simulink model "APPL_DriverFaultDetection"  (R2018b)
settings: configuration reference "CodeConfig_10_ms" (kept outside this file)
undefined symbols (not defined in the file): CAL_LockErrNoTime_30ms, CAL_ManualSwValid_90s, CAL_MotorHallInvalid_2s, CAL_MotorMaxRunTime_60s, CAL_MotorRelayErr_2s, CAL_MotorStall_750ms, D_DrSoftStopDef_B, D_DrSoftStopDef_F, D_DrSoftStopDef_H, D_DrSoftStopDef_L, D_Relay_DownBackFault, D_Relay_UpFrontFault, enSeatMoveCmd, FALSE, TRUE
libraries: DareLib x95, simulink x2
(part 3 of 3)

== stateflow chart APPL_DriverFaultDetection/LogicCtrl/HallError/HallErrorDetection ==
  note: #后期需要增加2F诊断判断20230510
  state MotorHallDetect
    state HeightHallError [parallel]
      settings: executionOrder=1
      state Judge
        ex:
        HeightHallTimer = 0;
        (default) -> (junction 16)
        MotorHallDetect.HeightHallError.Judge -> (junction 16) [order 1]
        (junction 16) -> (junction 19) [order 1] : /*2s超时检测*/
            | [CAL_MotorHallInvalid_2s > HeightHallTimer]
        (junction 19) -> (junction 178)
        (junction 16) -> (junction 30) [order 2] : {HeightHallTimer = CAL_MotorHallInvalid_2s;
            | HeightHallFault = 1;
            | Desc_HeightHallDTC = 1;}
        (junction 178) -> (junction 180) [order 1] : /* 粘连或无电机动作 */
            | [MtrCtrlFault_HeightUpVolt == MtrCtrlFault_HeightDownVolt ...
            | || enSeatMoveCmd.EN_NULL == MtrCtrlFault_HeightMotorCmd]
        (junction 178) -> (junction 162) [order 2] : {HeightHallTimer ++;}
        (junction 180) -> (junction 182) : {HeightHallTimer = 0;}
        (junction 162) -> (junction 30)
        (junction 182) -> (junction 162)
        (junction 30) -> (junction 21)
        (junction 21) -> (junction 23) [order 1] : /*霍尔计数变化*/
            | [hasChanged(MtrCtrlFault_HeightHallCnt)]
        (junction 21) -> (junction 28) [order 2]
        (junction 23) -> (junction 26) : {HeightHallTimer = 0;
            | HeightHallFault = 0;
            | Desc_HeightHallDTC = 0;}
        (junction 26) -> (junction 28)
      state Normal
        en:
        HeightHallFault = 0;
      state Init
        en:
        HeightHallFault = 0;
        Desc_HeightHallDTC = 0;
      (default) -> MotorHallDetect.HeightHallError.Normal
      MotorHallDetect.HeightHallError.Normal -> MotorHallDetect.HeightHallError.Judge [order 2] : /*有调节动作*/
          | [enSeatMoveCmd.EN_NULL != MtrCtrlFault_HeightMotorCmd]
      MotorHallDetect.HeightHallError.Judge -> MotorHallDetect.HeightHallError.Normal [order 2] : /* */
          | [(hasChanged(HeightSwCmd) ...
          | || enSeatMoveCmd.EN_NULL == HeightSwCmd) ...
          | && enSeatMoveCmd.EN_NULL == MtrCtrlFault_HeightMotorCmd]
      MotorHallDetect.HeightHallError.Judge -> MotorHallDetect.HeightHallError.Init [order 1] : /* 不满足前置条件 */
          | [FALSE == DrAdj_Dtc_HeatingMat1SC]
      MotorHallDetect.HeightHallError.Init -> MotorHallDetect.HeightHallError.Normal : /* 满足前置条件 */
          | [TRUE == DrAdj_Dtc_HeatingMat1SC]
      MotorHallDetect.HeightHallError.Normal -> MotorHallDetect.HeightHallError.Init [order 1] : /* 不满足前置条件 */
          | [FALSE == DrAdj_Dtc_HeatingMat1SC]
    state LengthHallError [parallel]
      settings: executionOrder=2
      state Normal
        en:
        LengthHallFault = 0;
      state Judge
        ex:
        LengthHallTimer = 0;
        (default) -> (junction 53)
        MotorHallDetect.LengthHallError.Judge -> (junction 53) [order 1]
        (junction 53) -> (junction 57) [order 1] : /*2s超时检测*/
            | [CAL_MotorHallInvalid_2s > LengthHallTimer]
        (junction 53) -> (junction 68) [order 2] : {LengthHallTimer = CAL_MotorHallInvalid_2s;
            | LengthHallFault = 1;
            | Desc_LengthHallDTC = 1;}
        (junction 57) -> (junction 185)
        (junction 185) -> (junction 187) [order 1] : /*粘连或无电机动作*/
            | [MtrCtrlFault_LengthForwardVolt == MtrCtrlFault_LengthBackwardVolt ...
            | || enSeatMoveCmd.EN_NULL == MtrCtrlFault_LengthMotorCmd]
        (junction 185) -> (junction 164) [order 2] : {LengthHallTimer ++;}
        (junction 187) -> (junction 189) : {LengthHallTimer = 0;}
        (junction 164) -> (junction 68)
        (junction 189) -> (junction 164)
        (junction 68) -> (junction 60)
        (junction 60) -> (junction 52) [order 1] : /*霍尔计数变化*/
            | [hasChanged(MtrCtrlFault_LengthHallCnt)]
        (junction 60) -> (junction 74) [order 2]
        (junction 52) -> (junction 62) : {LengthHallTimer = 0;
            | LengthHallFault = 0;
            | Desc_LengthHallDTC = 0;}
        (junction 62) -> (junction 74)
        (junction 74) -> (junction 64)
      state Init
        en:
        LengthHallFault = 0;
        Desc_LengthHallDTC = 0;
      (default) -> MotorHallDetect.LengthHallError.Normal
      MotorHallDetect.LengthHallError.Normal -> MotorHallDetect.LengthHallError.Judge [order 2] : /*有调节动作*/
          | [enSeatMoveCmd.EN_NULL != MtrCtrlFault_LengthMotorCmd]
      MotorHallDetect.LengthHallError.Judge -> MotorHallDetect.LengthHallError.Normal [order 2] : /*无调节动作*/
          | [(hasChanged(LengthSwCmd) ...
          | || enSeatMoveCmd.EN_NULL == LengthSwCmd) ...
          | && enSeatMoveCmd.EN_NULL == MtrCtrlFault_LengthMotorCmd]
      MotorHallDetect.LengthHallError.Judge -> MotorHallDetect.LengthHallError.Init [order 1] : /* 不满足前置条件 */
          | [FALSE == DrAdj_Dtc_HeatingMat1SC]
      MotorHallDetect.LengthHallError.Init -> MotorHallDetect.LengthHallError.Normal : /* 满足前置条件 */
          | [TRUE == DrAdj_Dtc_HeatingMat1SC]
      MotorHallDetect.LengthHallError.Normal -> MotorHallDetect.LengthHallError.Init [order 1] : /* 不满足前置条件 */
          | [FALSE == DrAdj_Dtc_HeatingMat1SC]
    state BackHallError [parallel]
      settings: executionOrder=3
      state Judge
        ex:
        BackHallTimer = 0;
        (default) -> (junction 87)
        MotorHallDetect.BackHallError.Judge -> (junction 87) [order 1]
        (junction 87) -> (junction 91) [order 1] : /*2s超时检测*/
            | [CAL_MotorHallInvalid_2s > BackHallTimer]
        (junction 87) -> (junction 102) [order 2] : {BackHallTimer = CAL_MotorHallInvalid_2s;
            | BackHallFault = 1;
            | Desc_BackHallDTC = 1;}
        (junction 91) -> (junction 192)
        (junction 192) -> (junction 194) [order 1] : /*粘连或无电机动作*/
            | [MtrCtrlFault_BackForwardVolt == MtrCtrlFault_BackBackwardVolt ...
            | || enSeatMoveCmd.EN_NULL == MtrCtrlFault_BackMotorCmd]
        (junction 192) -> (junction 166) [order 2] : {BackHallTimer ++;}
        (junction 194) -> (junction 196) : {BackHallTimer = 0;}
        (junction 166) -> (junction 102)
        (junction 196) -> (junction 166)
        (junction 102) -> (junction 94)
        (junction 94) -> (junction 86) [order 1] : /*霍尔计数变化*/
            | [hasChanged(MtrCtrlFault_BackHallCnt)]
        (junction 94) -> (junction 108) [order 2]
        (junction 86) -> (junction 96) : {BackHallTimer = 0;
            | BackHallFault = 0;
            | Desc_BackHallDTC = 0;}
        (junction 96) -> (junction 108)
        (junction 108) -> (junction 98)
      state Normal
        en:
        BackHallFault = 0;
      state Init
        en:
        BackHallFault = 0;
        Desc_BackHallDTC = 0;
      (default) -> MotorHallDetect.BackHallError.Normal
      MotorHallDetect.BackHallError.Normal -> MotorHallDetect.BackHallError.Judge [order 2] : /*有调节动作*/
          | [enSeatMoveCmd.EN_NULL != MtrCtrlFault_BackMotorCmd]
      MotorHallDetect.BackHallError.Judge -> MotorHallDetect.BackHallError.Normal [order 2] : /*无调节动作*/
          | [(hasChanged(BackSwCmd) ...
          | || enSeatMoveCmd.EN_NULL == BackSwCmd) ...
          | && enSeatMoveCmd.EN_NULL == MtrCtrlFault_BackMotorCmd]
      MotorHallDetect.BackHallError.Judge -> MotorHallDetect.BackHallError.Init [order 1] : /* 不满足前置条件 */
          | [FALSE == DrAdj_Dtc_HeatingMat1SC]
      MotorHallDetect.BackHallError.Init -> MotorHallDetect.BackHallError.Normal : /* 满足前置条件 */
          | [TRUE == DrAdj_Dtc_HeatingMat1SC]
      MotorHallDetect.BackHallError.Normal -> MotorHallDetect.BackHallError.Init [order 1] : /* 不满足前置条件 */
          | [FALSE == DrAdj_Dtc_HeatingMat1SC]
    state FrontHallError3 [parallel]
      settings: executionOrder=4
      state Judge
        ex:
        FrontHallTimer = 0;
        (default) -> (junction 121)
        MotorHallDetect.FrontHallError3.Judge -> (junction 121) [order 1]
        (junction 121) -> (junction 125) [order 1] : /*2s超时检测*/
            | [CAL_MotorHallInvalid_2s > FrontHallTimer]
        (junction 121) -> (junction 136) [order 2] : {FrontHallTimer = CAL_MotorHallInvalid_2s;
            | FrontHallFault = 1;
            | Desc_FrontHallDTC = 1;}
        (junction 125) -> (junction 199)
        (junction 199) -> (junction 201) [order 1] : /*粘连或无电机动作*/
            | [MtrCtrlFault_FrontUpVolt == MtrCtrlFault_FrontDownVolt ...
            | || enSeatMoveCmd.EN_NULL == MtrCtrlFault_FrontMotorCmd]
        (junction 199) -> (junction 169) [order 2] : {FrontHallTimer ++;}
        (junction 201) -> (junction 203) : {FrontHallTimer = 0;}
        (junction 169) -> (junction 136)
        (junction 203) -> (junction 169)
        (junction 136) -> (junction 128)
        (junction 128) -> (junction 120) [order 1] : /*霍尔计数变化*/
            | [hasChanged(MtrCtrlFault_FrontHallCnt)]
        (junction 128) -> (junction 142) [order 2]
        (junction 120) -> (junction 130) : {FrontHallTimer = 0;
            | FrontHallFault = 0;
            | Desc_FrontHallDTC = 0;}
        (junction 130) -> (junction 142)
        (junction 142) -> (junction 132)
      state Normal
        en:
        FrontHallFault = 0;
      state Init
        en:
        FrontHallFault = 0;
        Desc_FrontHallDTC = 0;
      (default) -> MotorHallDetect.FrontHallError3.Normal
      MotorHallDetect.FrontHallError3.Normal -> MotorHallDetect.FrontHallError3.Judge [order 1] : /*有调节动作*/
          | [enSeatMoveCmd.EN_NULL != MtrCtrlFault_FrontMotorCmd ...
          |  && EN_DrTwelveWayMotor == MtrCtrlFault_DrAdjustCfg]
      MotorHallDetect.FrontHallError3.Judge -> MotorHallDetect.FrontHallError3.Normal [order 2] : /*无调节动作*/
          | [((hasChanged(FrontSwCmd) ...
          | || enSeatMoveCmd.EN_NULL == FrontSwCmd) ...
          | && enSeatMoveCmd.EN_NULL == MtrCtrlFault_FrontMotorCmd) ...
          | || EN_DrTwelveWayMotor != MtrCtrlFault_DrAdjustCfg]
      MotorHallDetect.FrontHallError3.Init -> MotorHallDetect.FrontHallError3.Normal : /* 满足前置条件 */
          | [TRUE == DrAdj_Dtc_HeatingMat1SC]
      MotorHallDetect.FrontHallError3.Judge -> MotorHallDetect.FrontHallError3.Init [order 1] : /* 不满足前置条件 */
          | [FALSE == DrAdj_Dtc_HeatingMat1SC ...
          | || EN_DrTwelveWayMotor != MtrCtrlFault_DrAdjustCfg]
      MotorHallDetect.FrontHallError3.Normal -> MotorHallDetect.FrontHallError3.Init [order 2] : /* 不满足前置条件 */
          | [FALSE == DrAdj_Dtc_HeatingMat1SC]
  state Init
    en:
    HeightHallFault = 0;
    HeightHallTimer = 0;
    Desc_HeightHallDTC = 0;
    LengthHallFault = 0;
    LengthHallTimer = 0;
    Desc_LengthHallDTC = 0;
    BackHallFault = 0;
    BackHallTimer = 0;
    Desc_BackHallDTC = 0;
    FrontHallFault = 0;
    FrontHallTimer = 0;
    Desc_FrontHallDTC = 0;
  (default) -> Init
  Init -> MotorHallDetect : /* 有记忆功能 且非不可调节配置 */
      | [TRUE == MtrCtrlFault_DrMemoryCfg ...
      | && (EN_DrSixWayMotor == MtrCtrlFault_DrAdjustCfg ...
      |     || EN_DrTwelveWayMotor == MtrCtrlFault_DrAdjustCfg)]
  MotorHallDetect -> Init : /* 无记忆功能 ||不可调节配置 */
      | [TRUE != MtrCtrlFault_DrMemoryCfg ...
      | || (EN_DrSixWayMotor != MtrCtrlFault_DrAdjustCfg ...
      |     && EN_DrTwelveWayMotor != MtrCtrlFault_DrAdjustCfg)]
  data: HeightSwCmd input; LengthSwCmd input; BackSwCmd input; FrontSwCmd input; MtrCtrlFault_HeightUpVolt input; MtrCtrlFault_HeightDownVolt input; MtrCtrlFault_LengthForwardVolt input; MtrCtrlFault_LengthBackwardVolt input; Desc_HeightHallDTC output uint8 =0; Desc_LengthHallDTC output uint8 =0; Desc_BackHallDTC output uint8 =0; Desc_FrontHallDTC output uint8 =0; MtrCtrlFault_BackForwardVolt input; MtrCtrlFault_BackBackwardVolt input; MtrCtrlFault_FrontUpVolt input; MtrCtrlFault_FrontDownVolt input; HeightHallFault output uint8; MtrCtrlFault_HeightHallCnt input; MtrCtrlFault_LengthHallCnt input; MtrCtrlFault_BackHallCnt input; MtrCtrlFault_FrontHallCnt input; MtrCtrlFault_HeightMotorCmd input; MtrCtrlFault_LengthMotorCmd input; MtrCtrlFault_BackMotorCmd input; MtrCtrlFault_FrontMotorCmd input; HeightHallTimer local uint8; CAL_MotorHallInvalid_2s parameter; LengthHallTimer local uint8; LengthHallFault output uint8; BackHallTimer local uint8; BackHallFault output uint8; FrontHallTimer local uint8; FrontHallFault output uint8; FALSE parameter; TRUE parameter; DrAdj_Dtc_HeatingMat1SC local boolean =1; MtrCtrlFault_DrAdjustCfg input; MtrCtrlFault_DrMemoryCfg input

== stateflow chart APPL_DriverFaultDetection/LogicCtrl/StallError/StallErrorDetection ==
  state HeightStallError [parallel]
    settings: executionOrder=1
    state Judge
      ex:
      HeightStallTimer = 0;
      HeightStallNoTimer = 0;
      (default) -> (junction 16)
      HeightStallError.Judge -> (junction 16) [order 1]
      (junction 16) -> (junction 19) [order 1] : /*达到堵转电流 且无霍尔变化 */
          | [LocalHeightHallCnt == MtrCtrlFault_HeightHallCnt]
      (junction 19) -> (junction 187) [order 1] : [1 == MtrCtrlFault_HeightCurrentOverFlag]
      (junction 187) -> (junction 194) [order 1] : [CurrentOverTimer1 < 255]
      (junction 16) -> (junction 30) [order 2] : {HeightStallTimer = 0;
          | CurrentOverTimer1 = 0;}
      (junction 19) -> (junction 191) [order 2] : {CurrentOverTimer1 = 0;}
      (junction 187) -> (junction 189) [order 2]
      (junction 194) -> (junction 196) : /* 高度大电流计时器 - 启动电压不超过30ms*/
          | {CurrentOverTimer1 ++;}
      (junction 189) -> (junction 191)
      (junction 196) -> (junction 189)
      (junction 191) -> (junction 21)
      (junction 21) -> (junction 23) [order 1] : /*高度的堵转条件检测*/
          | [HeightStallTimer > CAL_MotorStall_750ms  ...
          | && CurrentOverTimer1 > 20]
      (junction 21) -> (junction 28) [order 2] : /* 高度无霍尔计时器*/
          | {HeightStallTimer ++;}
      (junction 23) -> (junction 26) : {HeightStallFault = 1;
          | HeightStallTimer = CAL_MotorStall_750ms;
          | HeightStallNoTimer = 0;}
      (junction 28) -> (junction 30)
      (junction 26) -> (junction 28)
      (junction 30) -> (junction 43) : {LocalHeightHallCnt = MtrCtrlFault_HeightHallCnt;}
      (junction 43) -> (junction 161) [order 1] : /*无调节动作 同时没有本地开关*/
          | [enSeatMoveCmd.EN_NULL == MtrCtrlFault_HeightMotorCmd ...
          | && enSeatMoveCmd.EN_NULL == HeightSwCmd]
      (junction 43) -> (junction 169) [order 2]
      (junction 161) -> (junction 163) : {HeightStallNoTimer++;}
      (junction 163) -> (junction 169)
      (junction 169) -> (junction 172)
    state Normal
      en:
      HeightStallFault = 0;
      CurrentOverTimer1 = 0;
    (default) -> HeightStallError.Normal
    HeightStallError.Normal -> HeightStallError.Judge : /*有调节动作*/
        | [enSeatMoveCmd.EN_NULL != MtrCtrlFault_HeightMotorCmd ...
        | && MtrCtrl_PowerModeStatus != enIgnSts.eCrank]
    HeightStallError.Judge -> HeightStallError.Normal [order 1] : /* 超过故障计时 或按键变化 */
        | [CAL_LockErrNoTime_30ms < HeightStallNoTimer ...
        | || hasChanged(HeightSwCmd) ...
        | || MtrCtrl_PowerModeStatus == enIgnSts.eCrank]
  state LengthStallError [parallel]
    settings: executionOrder=2
    state Judge
      ex:
      LengthStallTimer = 0;
      LengthStallNoTimer = 0;
      (default) -> (junction 53)
      LengthStallError.Judge -> (junction 53) [order 1]
      (junction 53) -> (junction 57) [order 1] : /*达到堵转电流 且无霍尔变化*/
          | [LocalLengthHallCnt == MtrCtrlFault_LengthHallCnt]
      (junction 57) -> (junction 210) [order 1] : [1 == MtrCtrlFault_LengthCurrentOverFlag]
      (junction 210) -> (junction 212) [order 1] : [CurrentOverTimer2 < 255]
      (junction 53) -> (junction 68) [order 2] : {LengthStallTimer = 0;
          | CurrentOverTimer2 = 0;}
      (junction 57) -> (junction 208) [order 2] : {CurrentOverTimer2 = 0;}
      (junction 210) -> (junction 216) [order 2]
      (junction 212) -> (junction 214) : /* 纵向大电流计时器*/
          | {CurrentOverTimer2 ++;}
      (junction 216) -> (junction 208)
      (junction 214) -> (junction 216)
      (junction 208) -> (junction 60)
      (junction 60) -> (junction 52) [order 1] : /*纵向的堵转条件检测*/
          | [LengthStallTimer > CAL_MotorStall_750ms  ...
          | && CurrentOverTimer2 > 20]
      (junction 60) -> (junction 74) [order 2] : {LengthStallTimer ++;}
      (junction 52) -> (junction 62) : {LengthStallTimer = CAL_MotorStall_750ms;
          | LengthStallFault = 1;
          | LengthStallNoTimer = 0;}
      (junction 74) -> (junction 68)
      (junction 62) -> (junction 74)
      (junction 68) -> (junction 78) : {LocalLengthHallCnt = MtrCtrlFault_LengthHallCnt;}
      (junction 78) -> (junction 80) [order 1] : /*无调节动作 同时没有本地开关*/
          | [enSeatMoveCmd.EN_NULL == MtrCtrlFault_LengthMotorCmd ...
          | && enSeatMoveCmd.EN_NULL == LengthSwCmd]
      (junction 78) -> (junction 70) [order 2]
      (junction 80) -> (junction 72) : {LengthStallNoTimer ++;}
      (junction 72) -> (junction 70)
      (junction 70) -> (junction 64)
    state Normal
      en:
      LengthStallFault = 0;
      CurrentOverTimer2 = 0;
    (default) -> LengthStallError.Normal
    LengthStallError.Normal -> LengthStallError.Judge : /*有调节动作*/
        | [enSeatMoveCmd.EN_NULL != MtrCtrlFault_LengthMotorCmd ...
        | && MtrCtrl_PowerModeStatus != enIgnSts.eCrank]
    LengthStallError.Judge -> LengthStallError.Normal [order 1] : /* 超过故障计时 或按键变化 */
        | [CAL_LockErrNoTime_30ms < LengthStallNoTimer ...
        | || hasChanged(LengthSwCmd) ...
        | || MtrCtrl_PowerModeStatus == enIgnSts.eCrank]
  state BackStallError [parallel]
    settings: executionOrder=3
    state Judge
      ex:
      BackStallTimer = 0;
      BackStallNoTimer = 0;
      (default) -> (junction 87)
      BackStallError.Judge -> (junction 87) [order 1]
      (junction 87) -> (junction 91) [order 1] : /* 无霍尔变化超时检测*/
          | [LocalBackHallCnt == MtrCtrlFault_BackHallCnt]
      (junction 91) -> (junction 223) [order 1] : [1 == MtrCtrlFault_BackCurrentOverFlag]
      (junction 223) -> (junction 228) [order 1] : [CurrentOverTimer3 < 255]
      (junction 87) -> (junction 102) [order 2] : {BackStallTimer = 0;
          | CurrentOverTimer3 = 0;}
      (junction 91) -> (junction 231) [order 2] : {CurrentOverTimer3 = 0;}
      (junction 223) -> (junction 229) [order 2]
      (junction 228) -> (junction 222) : /* 靠背大电流计时器*/
          | {CurrentOverTimer3 ++;}
      (junction 229) -> (junction 231)
      (junction 222) -> (junction 229)
      (junction 231) -> (junction 94)
      (junction 94) -> (junction 86) [order 1] : /*靠背的堵转条件检测*/
          | [BackStallTimer > CAL_MotorStall_750ms  ...
          | && CurrentOverTimer3 > 20]
      (junction 94) -> (junction 108) [order 2] : {BackStallTimer ++;}
      (junction 86) -> (junction 96) : {BackStallTimer = CAL_MotorStall_750ms;
          | BackStallFault = 1;
          | BackStallNoTimer = 0;}
      (junction 108) -> (junction 102)
      (junction 96) -> (junction 108)
      (junction 102) -> (junction 112) : {LocalBackHallCnt = MtrCtrlFault_BackHallCnt;}
      (junction 112) -> (junction 114) [order 1] : /*无调节动作 同时没有本地开关*/
          | [enSeatMoveCmd.EN_NULL == MtrCtrlFault_BackMotorCmd ...
          | && enSeatMoveCmd.EN_NULL == BackSwCmd]
      (junction 112) -> (junction 104) [order 2]
      (junction 114) -> (junction 106) : {BackStallNoTimer ++;}
      (junction 106) -> (junction 104)
      (junction 104) -> (junction 98)
    state Normal
      en:
      BackStallFault = 0;
      CurrentOverTimer3 = 0;
    (default) -> BackStallError.Normal
    BackStallError.Normal -> BackStallError.Judge : /*有调节动作*/
        | [enSeatMoveCmd.EN_NULL != MtrCtrlFault_BackMotorCmd ...
        | && MtrCtrl_PowerModeStatus != enIgnSts.eCrank]
    BackStallError.Judge -> BackStallError.Normal [order 1] : /* 超过故障计时 或按键变化 */
        | [CAL_LockErrNoTime_30ms < BackStallNoTimer ...
        | || hasChanged(BackSwCmd) ...
        | || MtrCtrl_PowerModeStatus == enIgnSts.eCrank]
  state FrontStallError [parallel]
    settings: executionOrder=4
    state Judge
      ex:
      FrontStallTimer = 0;
      FrontStallNoTimer = 0;
      (default) -> (junction 270)
      FrontStallError.Judge -> (junction 270) [order 1]
      (junction 270) -> (junction 271) [order 1] : /* 无霍尔变化超时检测*/
          | [LocalFrontHallCnt == MtrCtrlFault_FrontHallCnt]
      (junction 271) -> (junction 235) [order 1] : [1 ==  MtrCtrlFault_FrontCurrentOverFlag]
      (junction 235) -> (junction 262) [order 1] : [CurrentOverTimer4 < 255]
      (junction 270) -> (junction 276) [order 2] : {FrontStallTimer = 0;
          | CurrentOverTimer4 = 0;}
      (junction 271) -> (junction 260) [order 2] : {CurrentOverTimer4 = 0;}
      (junction 235) -> (junction 237) [order 2]
      (junction 262) -> (junction 265) : /* 靠背大电流计时器*/
          | {CurrentOverTimer4 ++;}
      (junction 237) -> (junction 260)
      (junction 265) -> (junction 237)
      (junction 260) -> (junction 263)
      (junction 263) -> (junction 273) [order 1] : /*靠背的堵转条件检测*/
          | [FrontStallTimer > CAL_MotorStall_750ms  ...
          | && CurrentOverTimer4 > 20]
      (junction 263) -> (junction 278) [order 2] : {FrontStallTimer ++;}
      (junction 273) -> (junction 253) : {FrontStallTimer = CAL_MotorStall_750ms;
          | FrontStallFault = 1;
          | FrontStallNoTimer = 0;}
      (junction 278) -> (junction 276)
      (junction 253) -> (junction 278)
      (junction 276) -> (junction 261) : {LocalFrontHallCnt = MtrCtrlFault_FrontHallCnt;}
      (junction 261) -> (junction 256) [order 1] : /*无调节动作 同时没有本地开关*/
          | [enSeatMoveCmd.EN_NULL == MtrCtrlFault_FrontMotorCmd ...
          | && enSeatMoveCmd.EN_NULL == FrontSwCmd]
      (junction 261) -> (junction 254) [order 2]
      (junction 256) -> (junction 255) : {FrontStallNoTimer ++;}
      (junction 255) -> (junction 254)
      (junction 254) -> (junction 258)
    state Normal
      en:
      FrontStallFault = 0;
      CurrentOverTimer4 = 0;
    (default) -> FrontStallError.Normal
    FrontStallError.Normal -> FrontStallError.Judge : /*有调节动作*/
        | [enSeatMoveCmd.EN_NULL != MtrCtrlFault_FrontMotorCmd ...
        | && MtrCtrl_PowerModeStatus != enIgnSts.eCrank]
    FrontStallError.Judge -> FrontStallError.Normal [order 1] : /* 超过故障计时 或按键变化 */
        | [CAL_LockErrNoTime_30ms < FrontStallNoTimer ...
        | || hasChanged(FrontSwCmd) ...
        | || MtrCtrl_PowerModeStatus == enIgnSts.eCrank]
  data: HeightSwCmd input; LengthSwCmd input; BackSwCmd input; HeightStallFault output uint8; FrontSwCmd input; MtrCtrlFault_HeightMotorCmd input; MtrCtrlFault_LengthMotorCmd input; MtrCtrlFault_BackMotorCmd input; MtrCtrlFault_FrontMotorCmd input; HeightStallTimer local uint8; CAL_MotorStall_750ms parameter; LengthStallTimer local uint8; LengthStallFault output uint8; BackStallTimer local uint8; BackStallFault output uint8; FrontStallTimer local uint8; FrontStallFault output uint8; MtrCtrlFault_HeightCurrentOverFlag input; MtrCtrlFault_LengthCurrentOverFlag input; MtrCtrlFault_BackCurrentOverFlag input; MtrCtrlFault_FrontCurrentOverFlag input; HeightStallNoTimer local uint8; LengthStallNoTimer local uint8; BackStallNoTimer local uint8; FrontStallNoTimer local uint8; CAL_LockErrNoTime_30ms parameter; MtrCtrlFault_HeightHallCnt input; MtrCtrlFault_LengthHallCnt input; MtrCtrlFault_BackHallCnt input; MtrCtrlFault_FrontHallCnt input; LocalLengthHallCnt local uint16; LocalHeightHallCnt local uint16; LocalBackHallCnt local uint16; LocalFrontHallCnt local uint16; MtrCtrl_PowerModeStatus input; CurrentOverTimer1 local uint8; CurrentOverTimer2 local uint8; CurrentOverTimer3 local uint8; CurrentOverTimer4 local uint8

== stateflow chart APPL_DriverFaultDetection/LogicCtrl/RelayError/MidRelayErrorDetection/CheckMidRelayFault1/RelayFault ==
  state Judge
    ex:
    MidRelayTimer = 0;
    (default) -> (junction 8)
    Judge -> (junction 8) [order 1]
    (junction 8) -> (junction 10) [order 1] : [CAL_MotorRelayErr_2s <= MidRelayTimer]
    (junction 8) -> (junction 14) [order 2] : {MidRelayTimer ++;}
    (junction 10) -> (junction 12) : {MidRelayTimer = CAL_MotorRelayErr_2s;}
    (junction 12) -> (junction 16) [order 1] : [enSeatMoveCmd.EN_UP_FORWARD != MotorCmd ...
        | && FALSE != UpForwardVolt]
    (junction 12) -> (junction 20) [order 2]
    (junction 16) -> (junction 18) : {MidRelayFault = D_Relay_UpFrontFault;}
    (junction 20) -> (junction 23) [order 1] : [enSeatMoveCmd.EN_DN_BACKWARD != MotorCmd ...
        | && FALSE != DownBackwardVolt]
    (junction 20) -> (junction 27) [order 2]
    (junction 23) -> (junction 25) : {MidRelayFault = D_Relay_DownBackFault;}
    (junction 14) -> (junction 27)
    (junction 25) -> (junction 27)
    (junction 18) -> (junction 25)
    (junction 27) -> (junction 31)
  state Normal
    en:
    MidRelayFault = FALSE;
    MidRelayTimer = 0;
  (default) -> Normal
  Normal -> Judge [order 1] : [/*没有输出命令但输出反馈有电压 满足前置条件*/
      | enSeatMoveCmd.EN_NULL == MotorCmd...
      | && (FALSE != UpForwardVolt...
      | || FALSE != DownBackwardVolt)]
  Normal -> Judge [order 2] : [/*输出命令向前/向上命令却有向后/向下电压 */
      | enSeatMoveCmd.EN_UP_FORWARD == MotorCmd...
      | &&  FALSE != DownBackwardVolt]
  Normal -> Judge [order 3] : [/*输出命令向后/向下命令却有向前/向上电压 */
      | enSeatMoveCmd.EN_DN_BACKWARD  == MotorCmd...
      | &&  FALSE != UpForwardVolt]
  Judge -> Normal [order 1] : [/*继电器粘连消失：
      |  1、没有控制开启命令，同时没有电压输出，认为继电器粘连消失
      |  2、控制开启命令，存在对应的电压输出，认为继电器粘连消失*/
      | (enSeatMoveCmd.EN_NULL == MotorCmd...
      | && FALSE == UpForwardVolt...
      | && FALSE == DownBackwardVolt) ...
      | || (enSeatMoveCmd.EN_UP_FORWARD == MotorCmd...
      | && TRUE == UpForwardVolt ...
      | && FALSE == DownBackwardVolt) ...
      | || (enSeatMoveCmd.EN_DN_BACKWARD == MotorCmd ...
      | && FALSE == UpForwardVolt ...
      | && TRUE == DownBackwardVolt) ]
  data: MotorCmd input; UpForwardVolt input; DownBackwardVolt input; MidRelayFault output uint8; CAL_MotorRelayErr_2s parameter; D_Relay_DownBackFault parameter; D_Relay_UpFrontFault parameter; FALSE parameter; TRUE parameter; MidRelayTimer output uint8

== stateflow chart APPL_DriverFaultDetection/LogicCtrl/RelayError/MidRelayErrorDetection/CheckMidRelayFault2/RelayFault ==
  state Judge
    ex:
    MidRelayTimer = 0;
    (default) -> (junction 8)
    Judge -> (junction 8) [order 1]
    (junction 8) -> (junction 10) [order 1] : [CAL_MotorRelayErr_2s <= MidRelayTimer]
    (junction 8) -> (junction 14) [order 2] : {MidRelayTimer ++;}
    (junction 10) -> (junction 12) : {MidRelayTimer = CAL_MotorRelayErr_2s;}
    (junction 12) -> (junction 16) [order 1] : [enSeatMoveCmd.EN_UP_FORWARD != MotorCmd ...
        | && FALSE != UpForwardVolt]
    (junction 12) -> (junction 20) [order 2]
    (junction 16) -> (junction 18) : {MidRelayFault = D_Relay_UpFrontFault;}
    (junction 20) -> (junction 23) [order 1] : [enSeatMoveCmd.EN_DN_BACKWARD != MotorCmd ...
        | && FALSE != DownBackwardVolt]
    (junction 20) -> (junction 27) [order 2]
    (junction 23) -> (junction 25) : {MidRelayFault = D_Relay_DownBackFault;}
    (junction 14) -> (junction 27)
    (junction 25) -> (junction 27)
    (junction 18) -> (junction 25)
    (junction 27) -> (junction 31)
  state Normal
    en:
    MidRelayFault = FALSE;
    MidRelayTimer = 0;
  (default) -> Normal
  Normal -> Judge [order 1] : [/*没有输出命令但输出反馈有电压 满足前置条件*/
      | enSeatMoveCmd.EN_NULL == MotorCmd...
      | && (FALSE != UpForwardVolt...
      | || FALSE != DownBackwardVolt)]
  Normal -> Judge [order 2] : [/*输出命令向前/向上命令却有向后/向下电压 */
      | enSeatMoveCmd.EN_UP_FORWARD == MotorCmd...
      | &&  FALSE != DownBackwardVolt]
  Normal -> Judge [order 3] : [/*输出命令向后/向下命令却有向前/向上电压 */
      | enSeatMoveCmd.EN_DN_BACKWARD  == MotorCmd...
      | &&  FALSE != UpForwardVolt]
  Judge -> Normal [order 1] : [/*继电器粘连消失：
      |  1、没有控制开启命令，同时没有电压输出，认为继电器粘连消失
      |  2、控制开启命令，存在对应的电压输出，认为继电器粘连消失*/
      | (enSeatMoveCmd.EN_NULL == MotorCmd...
      | && FALSE == UpForwardVolt...
      | && FALSE == DownBackwardVolt) ...
      | || (enSeatMoveCmd.EN_UP_FORWARD == MotorCmd...
      | && TRUE == UpForwardVolt ...
      | && FALSE == DownBackwardVolt) ...
      | || (enSeatMoveCmd.EN_DN_BACKWARD == MotorCmd ...
      | && FALSE == UpForwardVolt ...
      | && TRUE == DownBackwardVolt) ]
  data: MotorCmd input; UpForwardVolt input; DownBackwardVolt input; MidRelayFault output uint8; CAL_MotorRelayErr_2s parameter; D_Relay_DownBackFault parameter; D_Relay_UpFrontFault parameter; FALSE parameter; TRUE parameter; MidRelayTimer output uint8

== stateflow chart APPL_DriverFaultDetection/LogicCtrl/RelayError/MidRelayErrorDetection/CheckMidRelayFault3/RelayFault ==
  state Judge
    ex:
    MidRelayTimer = 0;
    (default) -> (junction 8)
    Judge -> (junction 8) [order 1]
    (junction 8) -> (junction 10) [order 1] : [CAL_MotorRelayErr_2s <= MidRelayTimer]
    (junction 8) -> (junction 14) [order 2] : {MidRelayTimer ++;}
    (junction 10) -> (junction 12) : {MidRelayTimer = CAL_MotorRelayErr_2s;}
    (junction 12) -> (junction 16) [order 1] : [enSeatMoveCmd.EN_UP_FORWARD != MotorCmd ...
        | && FALSE != UpForwardVolt]
    (junction 12) -> (junction 20) [order 2]
    (junction 16) -> (junction 18) : {MidRelayFault = D_Relay_UpFrontFault;}
    (junction 20) -> (junction 23) [order 1] : [enSeatMoveCmd.EN_DN_BACKWARD != MotorCmd ...
        | && FALSE != DownBackwardVolt]
    (junction 20) -> (junction 27) [order 2]
    (junction 23) -> (junction 25) : {MidRelayFault = D_Relay_DownBackFault;}
    (junction 14) -> (junction 27)
    (junction 25) -> (junction 27)
    (junction 18) -> (junction 25)
    (junction 27) -> (junction 31)
  state Normal
    en:
    MidRelayFault = FALSE;
    MidRelayTimer = 0;
  (default) -> Normal
  Normal -> Judge [order 1] : [/*没有输出命令但输出反馈有电压 满足前置条件*/
      | enSeatMoveCmd.EN_NULL == MotorCmd...
      | && (FALSE != UpForwardVolt...
      | || FALSE != DownBackwardVolt)]
  Normal -> Judge [order 2] : [/*输出命令向前/向上命令却有向后/向下电压 */
      | enSeatMoveCmd.EN_UP_FORWARD == MotorCmd...
      | &&  FALSE != DownBackwardVolt]
  Normal -> Judge [order 3] : [/*输出命令向后/向下命令却有向前/向上电压 */
      | enSeatMoveCmd.EN_DN_BACKWARD  == MotorCmd...
      | &&  FALSE != UpForwardVolt]
  Judge -> Normal [order 1] : [/*继电器粘连消失：
      |  1、没有控制开启命令，同时没有电压输出，认为继电器粘连消失
      |  2、控制开启命令，存在对应的电压输出，认为继电器粘连消失*/
      | (enSeatMoveCmd.EN_NULL == MotorCmd...
      | && FALSE == UpForwardVolt...
      | && FALSE == DownBackwardVolt) ...
      | || (enSeatMoveCmd.EN_UP_FORWARD == MotorCmd...
      | && TRUE == UpForwardVolt ...
      | && FALSE == DownBackwardVolt) ...
      | || (enSeatMoveCmd.EN_DN_BACKWARD == MotorCmd ...
      | && FALSE == UpForwardVolt ...
      | && TRUE == DownBackwardVolt) ]
  data: MotorCmd input; UpForwardVolt input; DownBackwardVolt input; MidRelayFault output uint8; CAL_MotorRelayErr_2s parameter; D_Relay_DownBackFault parameter; D_Relay_UpFrontFault parameter; FALSE parameter; TRUE parameter; MidRelayTimer output uint8

== stateflow chart APPL_DriverFaultDetection/LogicCtrl/MotorTimeOut/MotorTimeOutDetection ==
  state HeightAdjust [parallel]
    settings: executionOrder=1
    state Init
      en:
      HeightTimer = 0;
      (default) -> (junction 362)
      HeightAdjust.Init -> (junction 362) [order 1]
      (junction 362) -> (junction 365) [order 1] : /* 按键无效 */
          | [FALSE == HeightManualAdjSw]
      (junction 362) -> (junction 369) [order 2]
      (junction 365) -> (junction 367) : {HeightTimeOutFlag =FALSE;}
      (junction 367) -> (junction 369)
      (junction 369) -> (junction 372)
    state Action
      (default) -> (junction 25)
      HeightAdjust.Action -> (junction 25) [order 1]
      (junction 25) -> (junction 26) [order 1] : [HeightTimer < CAL_MotorMaxRunTime_60s]
      (junction 25) -> (junction 27) [order 2] : {HeightTimeOutFlag =TRUE;}
      (junction 26) -> (junction 28) : {HeightTimer++;}
      (junction 28) -> (junction 27)
      (junction 27) -> (junction 317)
    (default) -> HeightAdjust.Init
    HeightAdjust.Init -> HeightAdjust.Action [order 1] : [EN_NULL != HeightMotorCmd]
    HeightAdjust.Action -> HeightAdjust.Init [order 1] : [EN_NULL == HeightMotorCmd]
  state VerticalAdjust [parallel]
    settings: executionOrder=2
    state Init
      en:
      LengthTimer = 0;
      (default) -> (junction 383)
      VerticalAdjust.Init -> (junction 383) [order 1]
      (junction 383) -> (junction 378) [order 1] : /* 按键无效 */
          | [FALSE == LengthManualAdjSw]
      (junction 383) -> (junction 385) [order 2]
      (junction 378) -> (junction 381) : {LengthTimeOutFlag = FALSE;}
      (junction 381) -> (junction 385)
      (junction 385) -> (junction 375)
    state Action
      (default) -> (junction 38)
      VerticalAdjust.Action -> (junction 38) [order 1]
      (junction 38) -> (junction 32) [order 1] : [LengthTimer < CAL_MotorMaxRunTime_60s]
      (junction 38) -> (junction 33) [order 2] : {LengthTimeOutFlag = TRUE;}
      (junction 32) -> (junction 40) : {LengthTimer++;}
      (junction 40) -> (junction 33)
      (junction 33) -> (junction 320)
    (default) -> VerticalAdjust.Init
    VerticalAdjust.Init -> VerticalAdjust.Action [order 1] : /*高度、纵向电机没有命令或计时已到*/
        | [EN_NULL != LengthMotorCmd]
    VerticalAdjust.Action -> VerticalAdjust.Init [order 1] : [EN_NULL == LengthMotorCmd]
  state BackAdjust [parallel]
    settings: executionOrder=3
    state Init
      en:
      BackTimer = 0;
      (default) -> (junction 390)
      BackAdjust.Init -> (junction 390) [order 1]
      (junction 390) -> (junction 395) [order 1] : /* 按键无效 */
          | [FALSE == BackManualAdjSw]
      (junction 390) -> (junction 388) [order 2]
      (junction 395) -> (junction 392) : {BackTimeOutFlag = FALSE;}
      (junction 392) -> (junction 388)
      (junction 388) -> (junction 394)
    state Action
      (default) -> (junction 79)
      BackAdjust.Action -> (junction 79) [order 1]
      (junction 79) -> (junction 73) [order 1] : [BackTimer < CAL_MotorMaxRunTime_60s]
      (junction 79) -> (junction 74) [order 2] : {BackTimeOutFlag = TRUE;}
      (junction 73) -> (junction 81) : {BackTimer++;}
      (junction 81) -> (junction 74)
      (junction 74) -> (junction 340)
    (default) -> BackAdjust.Init
    BackAdjust.Init -> BackAdjust.Action [order 1] : /*高度、纵向、前部电机没有命令或计时已到*/
        | [EN_NULL != BackMotorCmd]
    BackAdjust.Action -> BackAdjust.Init [order 1] : [EN_NULL == BackMotorCmd]
  state FrontAngleAdjust [parallel]
    settings: executionOrder=4
    state Init
      en:
      FrontTimer = 0;
      (default) -> (junction 406)
      FrontAngleAdjust.Init -> (junction 406) [order 1]
      (junction 406) -> (junction 401) [order 1] : /* 按键无效 */
          | [FALSE == FrontManualAdjSw]
      (junction 406) -> (junction 403) [order 2]
      (junction 401) -> (junction 400) : {FrontTimeOutFlag = FALSE;}
      (junction 400) -> (junction 403)
      (junction 403) -> (junction 399)
    state Action
      (default) -> (junction 103)
      FrontAngleAdjust.Action -> (junction 103) [order 1]
      (junction 103) -> (junction 109) [order 1] : [FrontTimer < CAL_MotorMaxRunTime_60s]
      (junction 103) -> (junction 101) [order 2] : {FrontTimeOutFlag = TRUE;}
      (junction 109) -> (junction 98) : {FrontTimer++;}
      (junction 98) -> (junction 101)
      (junction 101) -> (junction 352)
    FrontAngleAdjust.Init -> FrontAngleAdjust.Action [order 1] : /*高度、纵向电机没有命令或计时已到*/
        | [EN_NULL != FrontMotorCmd]
    FrontAngleAdjust.Action -> FrontAngleAdjust.Init [order 1] : [EN_NULL == FrontMotorCmd]
  (default) -> FrontAngleAdjust.Init
  data: HeightMotorCmd input; LengthMotorCmd input; BackMotorCmd input; FrontMotorCmd input; EN_NULL input; BackTimer local uint16; FrontTimer local uint16; HeightTimer local uint16; LengthTimer local uint16; HeightTimeOutFlag output uint8; LengthTimeOutFlag output uint8; BackTimeOutFlag output uint8; FrontTimeOutFlag output uint8; CAL_MotorMaxRunTime_60s parameter; TRUE parameter; FALSE parameter; HeightManualAdjSw input; LengthManualAdjSw input; BackManualAdjSw input; FrontManualAdjSw input

== stateflow chart APPL_DriverFaultDetection/LogicCtrl/SoftStopPoint/SoftStopPointDetection ==
  state InputData [parallel]
    en:
    du:
    HeightSoftStopBufCnt = MtrCtrlFault_HeightSoftStopCnt;
    LengthSoftStopBufCnt = MtrCtrlFault_LengthSoftStopCnt;
    BackSoftStopBufCnt = MtrCtrlFault_BackSoftStopCnt;
    FrontSoftStopBufCnt = MtrCtrlFault_FrontSoftStopCnt;
    settings: executionOrder=1
  state DrAdj_SetHeightSoftStopCnt(Cnt) [function]
  state DrAdj_SetLengthSoftStopCnt(Cnt) [function]
  state HeightSoft [parallel]
    settings: executionOrder=2
    state LeftUpFront
      (default) -> (junction 55)
      HeightSoft.LeftUpFront -> (junction 55) [order 1]
      (junction 55) -> (junction 58) : {HeightSoftStopFault = enSeatMoveCmd.EN_NULL;}
      (junction 58) -> (junction 60) [order 1] : /* 超过最大软止点 */
          | [MtrCtrlFault_HeightHallCnt >= (MtrCtrlFault_HeightStopPosi + MtrCtrlFault_HeightMotorSize - D_DrSoftStopDef_H)]
      (junction 58) -> (junction 69) [order 2]
      (junction 60) -> (junction 67) : {HeightSoftStopBufCnt += 1;
          | HeightSoftStopFault = enSeatMoveCmd.EN_UP_FORWARD;
          | DrAdj_SetHeightSoftStopCnt(HeightSoftStopBufCnt);}
      (junction 67) -> (junction 69)
      (junction 69) -> (junction 87)
    state Init
      (default) -> (junction 91)
      HeightSoft.Init -> (junction 91) [order 1]
      (junction 91) -> (junction 94) [order 1] : /*超过计数无故障 */
          | [HeightSoftStopBufCnt >= MtrCtrlFault_MotorSoftStopCntMax]
      (junction 91) -> (junction 98) [order 2]
      (junction 94) -> (junction 96) : {HeightSoftStopFault = enSeatMoveCmd.EN_NULL;}
      (junction 96) -> (junction 98)
      (junction 98) -> (junction 101)
    state RightDnBack
      (default) -> (junction 82)
      HeightSoft.RightDnBack -> (junction 82) [order 1]
      (junction 82) -> (junction 85) : {HeightSoftStopFault = enSeatMoveCmd.EN_NULL;}
      (junction 85) -> (junction 83) [order 1] : /* 超过最小软止点 */
          | [MtrCtrlFault_HeightHallCnt <= (MtrCtrlFault_HeightStopPosi + D_DrSoftStopDef_H)]
      (junction 85) -> (junction 79) [order 2]
      (junction 83) -> (junction 78) : {HeightSoftStopBufCnt += 1;
          | HeightSoftStopFault = enSeatMoveCmd.EN_DN_BACKWARD;
          | DrAdj_SetHeightSoftStopCnt(HeightSoftStopBufCnt);}
      (junction 78) -> (junction 79)
      (junction 79) -> (junction 89)
    (default) -> HeightSoft.Init
    HeightSoft.Init -> HeightSoft.RightDnBack [order 2] : /* 已学习硬止点
        | 软止点计数小于 最大值
        | 有控制指令 */
        | [0 != MtrCtrlFault_HeightStopPosi ...
        | && 0xFFFF != MtrCtrlFault_HeightStopPosi ...
        | && HeightSoftStopBufCnt < MtrCtrlFault_MotorSoftStopCntMax ...
        | && MtrCtrlFault_HeightMotorCmd == enSeatMoveCmd.EN_DN_BACKWARD ...
        | && HeightSoftStopFault != enSeatMoveCmd.EN_DN_BACKWARD]
    HeightSoft.Init -> HeightSoft.LeftUpFront [order 1] : /* 已学习硬止点
        | 软止点计数小于 最大值
        | 有控制指令 */
        | [0 != MtrCtrlFault_HeightStopPosi ...
        | && 0xFFFF != MtrCtrlFault_HeightStopPosi ...
        | && HeightSoftStopBufCnt < MtrCtrlFault_MotorSoftStopCntMax ...
        | && MtrCtrlFault_HeightMotorCmd == enSeatMoveCmd.EN_UP_FORWARD ...
        | && HeightSoftStopFault != enSeatMoveCmd.EN_UP_FORWARD]
    HeightSoft.LeftUpFront -> HeightSoft.Init [order 1] : /*无控制指令 */
        | [MtrCtrlFault_HeightMotorCmd == enSeatMoveCmd.EN_NULL ...
        | || HeightSoftStopFault == enSeatMoveCmd.EN_UP_FORWARD]
    HeightSoft.RightDnBack -> HeightSoft.Init [order 1] : /*无控制指令 */
        | [MtrCtrlFault_HeightMotorCmd == enSeatMoveCmd.EN_NULL ...
        | || HeightSoftStopFault == enSeatMoveCmd.EN_DN_BACKWARD]
  state DrAdj_SetBackSoftStopCnt(Cnt) [function]
  state DrAdj_SetFrontSoftStopCnt(Cnt) [function]
  state LengthSoft [parallel]
    settings: executionOrder=3
    state LeftUpFront
      (default) -> (junction 124)
      LengthSoft.LeftUpFront -> (junction 124) [order 1]
      (junction 124) -> (junction 129) : {LengthSoftStopFault = enSeatMoveCmd.EN_NULL;}
      (junction 129) -> (junction 125) [order 1] : /* 超过最大软止点 */
          | [MtrCtrlFault_LengthHallCnt >= (MtrCtrlFault_LengthStopPosi + MtrCtrlFault_LengthMotorSize - D_DrSoftStopDef_L)]
      (junction 129) -> (junction 120) [order 2]
      (junction 125) -> (junction 119) : {LengthSoftStopBufCnt += 1;
          | LengthSoftStopFault = enSeatMoveCmd.EN_UP_FORWARD;
          | DrAdj_SetLengthSoftStopCnt(LengthSoftStopBufCnt);}
      (junction 119) -> (junction 120)
      (junction 120) -> (junction 145)
    state Init
      (default) -> (junction 143)
      LengthSoft.Init -> (junction 143) [order 1]
      (junction 143) -> (junction 136) [order 1] : /*超过计数无故障 */
          | [LengthSoftStopBufCnt >= MtrCtrlFault_MotorSoftStopCntMax]
      (junction 143) -> (junction 135) [order 2]
      (junction 136) -> (junction 149) : {LengthSoftStopFault = enSeatMoveCmd.EN_NULL;}
      (junction 149) -> (junction 135)
      (junction 135) -> (junction 138)
    state RightDnBack
      (default) -> (junction 103)
      LengthSoft.RightDnBack -> (junction 103) [order 1]
      (junction 103) -> (junction 111) : {LengthSoftStopFault = enSeatMoveCmd.EN_NULL;}
      (junction 111) -> (junction 112) [order 1] : /* 超过最小软止点 */
          | [MtrCtrlFault_LengthHallCnt <= (MtrCtrlFault_LengthStopPosi + D_DrSoftStopDef_L)]
      (junction 111) -> (junction 108) [order 2]
      (junction 112) -> (junction 105) : {LengthSoftStopBufCnt += 1;
          | LengthSoftStopFault = enSeatMoveCmd.EN_DN_BACKWARD;
          | DrAdj_SetLengthSoftStopCnt(LengthSoftStopBufCnt);}
      (junction 105) -> (junction 108)
      (junction 108) -> (junction 140)
    (default) -> LengthSoft.Init
    LengthSoft.Init -> LengthSoft.RightDnBack [order 2] : /* 已学习硬止点
        | 软止点计数小于 最大值
        | 有控制指令 */
        | [0 != MtrCtrlFault_LengthStopPosi ...
        | && 0xFFFF != MtrCtrlFault_LengthStopPosi ...
        | && LengthSoftStopBufCnt < MtrCtrlFault_MotorSoftStopCntMax ...
        | && MtrCtrlFault_LengthMotorCmd == enSeatMoveCmd.EN_DN_BACKWARD ...
        | && LengthSoftStopFault != enSeatMoveCmd.EN_DN_BACKWARD]
    LengthSoft.Init -> LengthSoft.LeftUpFront [order 1] : /* 已学习硬止点
        | 软止点计数小于 最大值
        | 有控制指令 */
        | [0 != MtrCtrlFault_LengthStopPosi ...
        | && 0xFFFF != MtrCtrlFault_LengthStopPosi ...
        | && LengthSoftStopBufCnt < MtrCtrlFault_MotorSoftStopCntMax ...
        | && MtrCtrlFault_LengthMotorCmd == enSeatMoveCmd.EN_UP_FORWARD ...
        | && LengthSoftStopFault != enSeatMoveCmd.EN_UP_FORWARD]
    LengthSoft.LeftUpFront -> LengthSoft.Init [order 1] : /*无控制指令 */
        | [MtrCtrlFault_LengthMotorCmd == enSeatMoveCmd.EN_NULL ...
        | || LengthSoftStopFault == enSeatMoveCmd.EN_UP_FORWARD]
    LengthSoft.RightDnBack -> LengthSoft.Init [order 1] : /*无控制指令 */
        | [MtrCtrlFault_LengthMotorCmd == enSeatMoveCmd.EN_NULL ...
        | || LengthSoftStopFault == enSeatMoveCmd.EN_DN_BACKWARD]
  state BackSoft [parallel]
    settings: executionOrder=4
    state LeftUpFront
      (default) -> (junction 181)
      BackSoft.LeftUpFront -> (junction 181) [order 1]
      (junction 181) -> (junction 185) : {BackSoftStopFault = enSeatMoveCmd.EN_NULL;}
      (junction 185) -> (junction 156) [order 1] : /* 超过最大软止点 */
          | [MtrCtrlFault_BackHallCnt >= (MtrCtrlFault_BackStopPosi + MtrCtrlFault_BackMotorSize - D_DrSoftStopDef_B)]
      (junction 185) -> (junction 186) [order 2]
      (junction 156) -> (junction 188) : {BackSoftStopBufCnt += 1;
          | BackSoftStopFault = enSeatMoveCmd.EN_UP_FORWARD;
          | DrAdj_SetBackSoftStopCnt(BackSoftStopBufCnt);}
      (junction 188) -> (junction 186)
      (junction 186) -> (junction 163)
    state Init
      (default) -> (junction 170)
      BackSoft.Init -> (junction 170) [order 1]
      (junction 170) -> (junction 158) [order 1] : /*超过计数无故障 */
          | [BackSoftStopBufCnt >= MtrCtrlFault_MotorSoftStopCntMax]
      (junction 170) -> (junction 191) [order 2]
      (junction 158) -> (junction 176) : {BackSoftStopFault = enSeatMoveCmd.EN_NULL;}
      (junction 176) -> (junction 191)
      (junction 191) -> (junction 193)
    state RightDnBack
      (default) -> (junction 184)
      BackSoft.RightDnBack -> (junction 184) [order 1]
      (junction 184) -> (junction 179) : {BackSoftStopFault = enSeatMoveCmd.EN_NULL;}
      (junction 179) -> (junction 177) [order 1] : /* 超过最小软止点 */
          | [MtrCtrlFault_BackHallCnt <= (MtrCtrlFault_BackStopPosi + D_DrSoftStopDef_B)]
      (junction 179) -> (junction 168) [order 2]
      (junction 177) -> (junction 196) : {BackSoftStopBufCnt += 1;
          | BackSoftStopFault = enSeatMoveCmd.EN_DN_BACKWARD;
          | DrAdj_SetBackSoftStopCnt(BackSoftStopBufCnt);}
      (junction 196) -> (junction 168)
      (junction 168) -> (junction 161)
    (default) -> BackSoft.Init
    BackSoft.Init -> BackSoft.RightDnBack [order 2] : /* 已学习硬止点
        | 软止点计数小于 最大值
        | 有控制指令 */
        | [0 != MtrCtrlFault_BackStopPosi ...
        | && 0xFFFF != MtrCtrlFault_BackStopPosi ...
        | && BackSoftStopBufCnt < MtrCtrlFault_MotorSoftStopCntMax ...
        | && MtrCtrlFault_BackMotorCmd == enSeatMoveCmd.EN_DN_BACKWARD ...
        | && BackSoftStopFault != enSeatMoveCmd.EN_DN_BACKWARD]
    BackSoft.Init -> BackSoft.LeftUpFront [order 1] : /* 已学习硬止点
        | 软止点计数小于 最大值
        | 有控制指令 */
        | [0 != MtrCtrlFault_BackStopPosi ...
        | && 0xFFFF != MtrCtrlFault_BackStopPosi ...
        | && BackSoftStopBufCnt < MtrCtrlFault_MotorSoftStopCntMax ...
        | && MtrCtrlFault_BackMotorCmd == enSeatMoveCmd.EN_UP_FORWARD ...
        | && BackSoftStopFault != enSeatMoveCmd.EN_UP_FORWARD]
    BackSoft.LeftUpFront -> BackSoft.Init [order 1] : /*无控制指令 */
        | [MtrCtrlFault_BackMotorCmd == enSeatMoveCmd.EN_NULL ...
        | || BackSoftStopFault == enSeatMoveCmd.EN_UP_FORWARD]
    BackSoft.RightDnBack -> BackSoft.Init [order 1] : /*无控制指令 */
        | [MtrCtrlFault_BackMotorCmd == enSeatMoveCmd.EN_NULL ...
        | || BackSoftStopFault == enSeatMoveCmd.EN_DN_BACKWARD]
  state FrontSoft [parallel]
    settings: executionOrder=5
    state LeftUpFront
      (default) -> (junction 207)
      FrontSoft.LeftUpFront -> (junction 207) [order 1]
      (junction 207) -> (junction 203) : {FrontSoftStopFault = enSeatMoveCmd.EN_NULL;}
      (junction 203) -> (junction 228) [order 1] : /* 超过最大软止点 */
          | [MtrCtrlFault_FrontHallCnt >= (MtrCtrlFault_FrontStopPosi + MtrCtrlFault_FrontMotorSize - D_DrSoftStopDef_F)]
      (junction 203) -> (junction 202) [order 2]
      (junction 228) -> (junction 226) : {FrontSoftStopBufCnt += 1;
          | FrontSoftStopFault = enSeatMoveCmd.EN_UP_FORWARD;
          | DrAdj_SetFrontSoftStopCnt(FrontSoftStopBufCnt);}
      (junction 226) -> (junction 202)
      (junction 202) -> (junction 223)
    state Init
      (default) -> (junction 218)
      FrontSoft.Init -> (junction 218) [order 1]
      (junction 218) -> (junction 230) [order 1] : /*超过计数无故障 */
          | [FrontSoftStopBufCnt >= MtrCtrlFault_MotorSoftStopCntMax]
      (junction 218) -> (junction 250) [order 2]
      (junction 230) -> (junction 212) : {FrontSoftStopFault = enSeatMoveCmd.EN_NULL;}
      (junction 212) -> (junction 250)
      (junction 250) -> (junction 234)
    state RightDnBack
      (default) -> (junction 204)
      FrontSoft.RightDnBack -> (junction 204) [order 1]
      (junction 204) -> (junction 209) : {FrontSoftStopFault = enSeatMoveCmd.EN_NULL;}
      (junction 209) -> (junction 210) [order 1] : /* 超过最小软止点 */
          | [MtrCtrlFault_FrontHallCnt <= (MtrCtrlFault_FrontStopPosi + D_DrSoftStopDef_F)]
      (junction 209) -> (junction 244) [order 2]
      (junction 210) -> (junction 235) : {FrontSoftStopBufCnt += 1;
          | FrontSoftStopFault = enSeatMoveCmd.EN_DN_BACKWARD;
          | DrAdj_SetFrontSoftStopCnt(FrontSoftStopBufCnt);}
      (junction 235) -> (junction 244)
      (junction 244) -> (junction 222)
    (default) -> FrontSoft.Init
    FrontSoft.Init -> FrontSoft.RightDnBack [order 1] : /* 已学习硬止点
        | 软止点计数小于 最大值
        | 有控制指令 */
        | [0 != MtrCtrlFault_FrontStopPosi ...
        | && 0xFFFF != MtrCtrlFault_FrontStopPosi ...
        | && FrontSoftStopBufCnt < MtrCtrlFault_MotorSoftStopCntMax ...
        | && MtrCtrlFault_FrontMotorCmd == enSeatMoveCmd.EN_DN_BACKWARD ...
        | && FrontSoftStopFault != enSeatMoveCmd.EN_DN_BACKWARD]
    FrontSoft.Init -> FrontSoft.LeftUpFront [order 2] : /* 已学习硬止点
        | 软止点计数小于 最大值
        | 有控制指令 */
        | [0 != MtrCtrlFault_FrontStopPosi ...
        | && 0xFFFF != MtrCtrlFault_FrontStopPosi ...
        | && FrontSoftStopBufCnt < MtrCtrlFault_MotorSoftStopCntMax ...
        | && MtrCtrlFault_FrontMotorCmd == enSeatMoveCmd.EN_UP_FORWARD ...
        | && FrontSoftStopFault != enSeatMoveCmd.EN_UP_FORWARD]
    FrontSoft.LeftUpFront -> FrontSoft.Init [order 1] : /*无控制指令 */
        | [MtrCtrlFault_FrontMotorCmd == enSeatMoveCmd.EN_NULL ...
        | || FrontSoftStopFault == enSeatMoveCmd.EN_UP_FORWARD]
    FrontSoft.RightDnBack -> FrontSoft.Init [order 1] : /*无控制指令 */
        | [MtrCtrlFault_FrontMotorCmd == enSeatMoveCmd.EN_NULL ...
        | || FrontSoftStopFault == enSeatMoveCmd.EN_DN_BACKWARD]
  data: Cnt function_input; Cnt function_input; Cnt function_input; Cnt function_input; MtrCtrlFault_HeightMotorCmd input; MtrCtrlFault_LengthMotorCmd input; MtrCtrlFault_BackMotorCmd input; MtrCtrlFault_FrontMotorCmd input; MtrCtrlFault_MotorSoftStopCntMax input; MtrCtrlFault_HeightSoftStopCnt input; MtrCtrlFault_LengthSoftStopCnt input; MtrCtrlFault_BackSoftStopCnt input; MtrCtrlFault_FrontSoftStopCnt input; MtrCtrlFault_HeightStopPosi input; MtrCtrlFault_LengthStopPosi input; MtrCtrlFault_BackStopPosi input; MtrCtrlFault_FrontStopPosi input; HeightSoftStopFault output uint8; LengthSoftStopFault output uint8; BackSoftStopFault output uint8; FrontSoftStopFault output uint8; MtrCtrlFault_HeightMotorSize input; MtrCtrlFault_LengthMotorSize input; MtrCtrlFault_BackMotorSize input; MtrCtrlFault_FrontMotorSize input; MtrCtrlFault_HeightHallCnt input; MtrCtrlFault_LengthHallCnt input; MtrCtrlFault_BackHallCnt input; MtrCtrlFault_FrontHallCnt input; HeightSoftStopBufCnt local uint8; LengthSoftStopBufCnt local uint8; BackSoftStopBufCnt local uint8; FrontSoftStopBufCnt local uint8; FALSE parameter; TRUE parameter; D_DrSoftStopDef_B parameter; D_DrSoftStopDef_L parameter; D_DrSoftStopDef_H parameter; D_DrSoftStopDef_F parameter

== stateflow chart APPL_DriverFaultDetection/LogicCtrl/AdheAndEffec/SwitchErrorDetection/TimeDiffTs/Chart ==
  (default) -> (junction 3)
  (junction 3) -> (junction 5)
  (junction 5) -> (junction 7) [order 1] : /* 入参比当前大 */
      | [lastTs > Ts]
  (junction 5) -> (junction 13) [order 2] : {OutTs = Ts - lastTs;}
  (junction 7) -> (junction 11) : {OutTs = 0xFFFFFFFF - lastTs + Ts +1;}
  (junction 11) -> (junction 13)
  (junction 13) -> (junction 17)
  data: lastTs input uint32; Ts input uint32; OutTs output uint32
